simulink model "AM5_1_spec"  (R2020b)
settings: Solver=VariableStepDiscrete  StartTime=0.0  StopTime=2  MaxStep=1/800  RelTol=1e-3
settings Model: Creator=seojoon  LastModifiedBy=seojoon

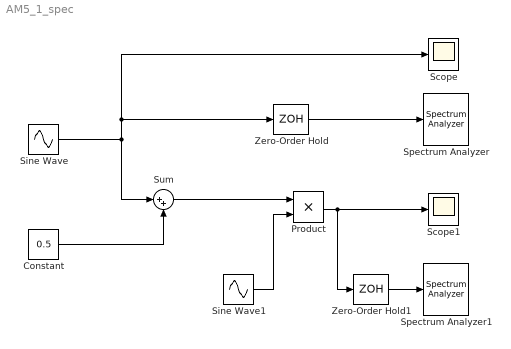
== system AM5_1_spec ==
  Constant : Constant  Value=0.5
  Product : Product
  Scope : Scope
  Scope1 : Scope
  Sine Wave : Sin  Amplitude=2  Frequency=2*pi*5  SampleTime=0
  Sine Wave1 : Sin  Frequency=2*pi*50  Phase=pi/2  SampleTime=0
  Spectrum Analyzer : SpectrumAnalyzer
  Spectrum Analyzer1 : SpectrumAnalyzer
  Sum : Sum  Inputs=|++
  Zero-Order Hold : ZeroOrderHold  SampleTime=1/2000
  Zero-Order Hold1 : ZeroOrderHold  SampleTime=1/2000
  wires:
  Sine Wave/1 -> Sum/1, Scope/1, Zero-Order Hold/1
  Constant/1 -> Sum/2
  Sum/1 -> Product/1
  Sine Wave1/1 -> Product/2
  Product/1 -> Zero-Order Hold1/1, Scope1/1
  Zero-Order Hold/1 -> Spectrum Analyzer/1
  Zero-Order Hold1/1 -> Spectrum Analyzer1/1
